simulink model "PD"  (R2018b)
settings: Solver=VariableStepAuto  StartTime=0.0  StopTime=10.0  MaxStep=0.01  MinStep=0.001  RelTol=1e-3
settings Model: Creator=Shubhi  LastModifiedBy=Shubhi
settings SolverCC: InitialStep=0.001  MaxConsecutiveMinStep=1000  ZeroCrossAlgorithm=Adaptive

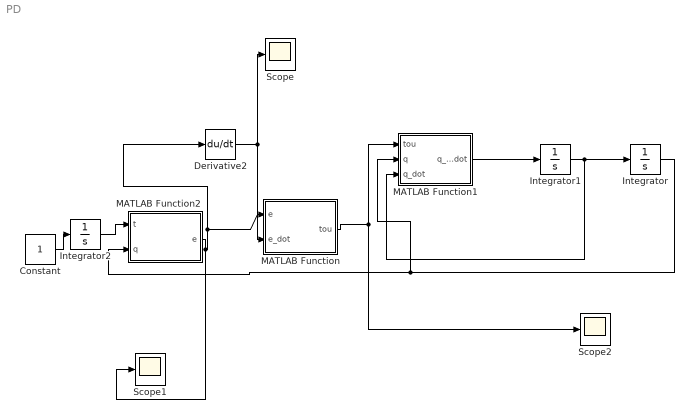
== system PD ==
  Constant : Constant
  Derivative2 : Derivative
  Integrator : Integrator  InitialCondition=[0;0]
  Integrator1 : Integrator  InitialCondition=[0;0]
  Integrator2 : Integrator
  MATLAB Function : MATLAB Function  TreatAsAtomicUnit=on
  MATLAB Function1 : MATLAB Function  TreatAsAtomicUnit=on
  MATLAB Function2 : MATLAB Function  TreatAsAtomicUnit=on
  Scope : Scope
  Scope1 : Scope
  Scope2 : Scope
  wires:
  MATLAB Function/1(tou) -> Scope2/1, MATLAB Function1/1(tou)
  MATLAB Function1/1(q_double_dot) -> Integrator1/1
  Integrator1/1 -> MATLAB Function1/3(q_dot), Integrator/1
  Integrator/1 -> MATLAB Function1/2(q), MATLAB Function2/2(q)
  Constant/1 -> Integrator2/1
  Integrator2/1 -> MATLAB Function2/1(t)
  MATLAB Function2/1(e) -> Scope1/1, Derivative2/1, MATLAB Function/1(e)
  Derivative2/1 -> Scope/1, MATLAB Function/2(e_dot)

== matlab function PD/MATLAB Function1 ==
  data: tou input; q input; q_double_dot output; q_dot input
function q_double_dot = fcn(tou,q,q_dot)

m1=3.473;
m2=0.196;
a1=1;  
a2=1;
g=9.81;
f1=5.3;
f2=1.1;

M=[(m1+m2)*a1*a1+m2*a2*a2+2*m2*a1*a2*cos(q(2)),m2*a2*a2+m2*a1*a2*cos(q(2));m2*a2*a2+m2*a1*a2*cos(q(2)),m2*a2*a2];  

V=[-m2*a1*a2*(2* q_dot(1)*q_dot(2)+q_dot(2)*q_dot(2))*sin(q(2));m2*a1*a2*q(1)*q(1)*sin(q(2))];

F=[f1,0;0,f2];

G=[(m1+m2)*g*a1*cos(q(1))+m2*g*a2*cos(q(1)+q(2)); m2*g*a2*cos(q(1)+q(2))];

q_double_dot=inv(M)*(tou-G-V-F*q_dot);

== matlab function PD/MATLAB Function ==
  data: tou output; e input; e_dot input
function tou =  fcn(e,e_dot)  
  
Kp=[200,10;10,200];
Kd=[200,10;10,200];

tou = -Kp*e-Kd*e_dot;

== matlab function PD/MATLAB Function2 ==
  data: t input; q input; e output
function e=fcn(t,q) 

qd=[pi/3+pi/6*sin(t);pi/4+pi/6*cos(t)]; 

e=q-qd;
